simulink model "MARCH_v1_5_stairs"  (R2016a)
settings: Solver=FixedStepDiscrete  StartTime=0.0  StopTime=inf  FixedStep=0.001  RelTol=1e-3
InitFcn:
  | % Change dir to model location
  | cd(fileparts(which(bdroot)));
  | 
  | init_model
  | initialize_model_testingBlocks
StartFcn:
  | cd(fileparts(which(bdroot)));
StopFcn:
  | cd(fileparts(which(bdroot)));
model workspace (MAT data in the model file):
  localValue = 1
  targetValue = 0
undefined symbols (not defined in the file or in its folder): Hip_HAA, Left_Leg, Right_Leg
libraries: xpcethercatlib x71, slrtlib x7, simulink x1, aerolibanimutils x1, dspnetwork x1
(part 3 of 3)

== matlab function MARCH_v1_5_stairs/Input Device/Generate random block signal safety/Saturation3  ==
  data: u input; y output
function y = fcn(u)

min = 0.1;
max = 0.3;

if u <= min
    y = min;
elseif u >= max;
    y = max;
else
    y = u;
end

== matlab function MARCH_v1_5_stairs/Input Device/Generate random block signal safety/Saturation4 ==
  data: u input; y output
function y = fcn(u)

min = 0.5;
max = 1.2;

if u <= min
    y = min;
elseif u >= max;
    y = max;
else
    y = u;
end

== matlab function MARCH_v1_5_stairs/Input Device/Generate random block signal trigger/Create peak1/Greater than 0 ==
  data: peak input; signal output
function signal  = fcn(peak)


if peak >= 0
    signal = peak;
else
    signal = 0;
    
    
end

== matlab function MARCH_v1_5_stairs/Input Device/Generate random block signal trigger/Create peak2/Greater than 0 ==
  data: peak input; signal output
function signal  = fcn(peak)


if peak >= 0
    signal = peak;
else
    signal = 0;
    
    
end

== matlab function MARCH_v1_5_stairs/Input Device/Generate random block signal trigger/Create peak3/Greater than 0 ==
  data: peak input; signal output
function signal  = fcn(peak)


if peak >= 0
    signal = peak;
else
    signal = 0;
    
    
end

== matlab function MARCH_v1_5_stairs/Input Device/Generate random block signal trigger/Rand. Block Func. Gen.1 ==
  data: u input; delayDurationInp input; blockDurationInp input; output output
function output  = fcn(u, delayDurationInp, blockDurationInp)

%% initialize the variable
persistent delayDuration blockDuration

if(isempty(blockDuration)||isempty(delayDuration))
    blockDuration = 0;
    delayDuration = 0;
    output = 0;
end

%% check if the delay and the block are done

doneDelay = (delayDuration <= 0);
doneBlock = (blockDuration <= 0);
done = (doneDelay && doneBlock);



%% Create delay and Block

if (u == 0 && done)
    output = 0;
elseif u == 1
    delayDuration = floor(1000*delayDurationInp);
    output = 0;
elseif not(doneDelay)
    delayDuration = delayDuration - 1;
    output = 0;
    if delayDuration == 0
        blockDuration = floor(1000*blockDurationInp);
        output = 1;
    end
elseif not(doneBlock)
    blockDuration = blockDuration - 1;
    output = 1;
else
    output = -1;
end


end

== matlab function MARCH_v1_5_stairs/Input Device/Generate random block signal trigger/Rand. Block Func. Gen.4 ==
  data: delayDurationInp input; blockDurationInp input; u input; output output
function output   = fcn(delayDurationInp, blockDurationInp, u)

%% initialize the variable
persistent delayDuration blockDuration

if(isempty(blockDuration)||isempty(delayDuration))
    blockDuration = 0;
    delayDuration = 0;
    output = 0;
end



%% check if the delay and the block are done

doneDelay = (delayDuration <= 0);
doneBlock = (blockDuration <= 0);
done = (doneDelay && doneBlock);



%% Create delay and Block

if (u == 0 && done)
    output = 0;
elseif u == 1
    delayDuration = floor(1000*delayDurationInp);
    output = 0;
elseif not(doneDelay)
    delayDuration = delayDuration - 1;
    output = 0;
    if delayDuration == 0
        blockDuration = floor(1000*blockDurationInp);
        output = 1;
    end
elseif not(doneBlock)
    blockDuration = blockDuration - 1;
    output = 1;
else
    output = -1;
end


end

== matlab function MARCH_v1_5_stairs/Input Device/Generate random block signal trigger/Saturation 2 ==
  data: u input; y output
function y = fcn(u)

min = 0.5;
max = 1.2;

if u <= min
    y = min;
elseif u >= max;
    y = max;
else
    y = u;
end

== matlab function MARCH_v1_5_stairs/Input Device/Generate random block signal trigger/Saturation1 ==
  data: u input; y output
function y = fcn(u)

min = 0.1;
max = 0.3;

if u <= min
    y = min;
elseif u >= max;
    y = max;
else
    y = u;
end

== matlab function MARCH_v1_5_stairs/Input Device/Generate random block signal trigger/Saturation3  ==
  data: u input; y output
function y = fcn(u)

min = 0.1;
max = 0.3;

if u <= min
    y = min;
elseif u >= max;
    y = max;
else
    y = u;
end

== matlab function MARCH_v1_5_stairs/Input Device/Generate random block signal trigger/Saturation4 ==
  data: u input; y output
function y = fcn(u)

min = 0.5;
max = 1.2;

if u <= min
    y = min;
elseif u >= max;
    y = max;
else
    y = u;
end

== matlab function MARCH_v1_5_stairs/Controllers/SitDown/Trajectory ==
  data: done output; q output; action input; q_i input size=[1 6]; q_f input; debugIn input
function [done,q] = fcn(action,q_i, q_f,debugIn)
%#codegen

persistent r splineCtrl i q_t n kneeDelay;

%% Initialize all variables
if(isempty(splineCtrl))
    splineCtrl = splineController();
end

if(isempty(r))
    % Get frequency of the model
    r = robotics();
    
end

if(isempty(q_t))
    q_t = [0 0 0 0 0 0];
    kneeDelay = [0 0];
end

if(isempty(i))
    i = 0;
    n = 0;
end


%% Logic
done = 0;

% Run sitdown procedure
if(n == 0 && i == 0)
    % Calculate final position based on robotics parameters
%     r.setTorsoHeight(debugIn);
%     r.refresh();
%     r.inverseKinematics();
%     q_f = r.q;
    
    splineCtrl.samples = 6500;
    q_t = splineCtrl.getJointTrajectory(q_i,q_f);

    % The hip rotation will play back halfway through the samples
    kneeDelay = splineCtrl.getCustomEaseTimeCurve(0.2,1);
    
    i = i+1;
    %q_t = splineCtrl.ease(q_t);
end

% Move hip backwards
if(n == 1 && i == 0)
    q_ff = [0 -1.80 q_f(3) 0 -1.80 q_f(6)];
    splineCtrl.samples = 1500;
    q_t = splineCtrl.getJointTrajectory(q_f,q_ff);
   
    i = i+1;
end


q = q_t(i,:);

% Slow down the knee trajectory only when standing up
if(n == 0)
    q(3) = splineCtrl.easeTrajectory(q_t(:,3),i,kneeDelay);
    q(6) = splineCtrl.easeTrajectory(q_t(:,6),i,kneeDelay);
end

if(i < length(q_t))
    i = i+1;
else
    if(n == 0)
        % Reset iterator
        i = 0;
        n = 1;
    else
        done = 1;
    end
end

end
